simulink model "sk_QR_Balanced"  (Simulink 9.0)
settings: Solver=ode45  StartTime=0.0  StopTime=T_sim  MaxStep=1e-3  RelTol=1e-3  EnableMultiTasking=on
values from neighbouring files (symbols this model uses):
  Tm = 1e-3    (= 0.001)    [Ejecucion.m]
settings Model: Creator=Isa  LastModifiedBy=Raúl  ExtModeTrigMode=oneshot  ExtModeArmWhenConnect=off
settings DataIOCC: SignalLoggingSaveFormat=ModelDataLogs
settings OptimizationCC: BlockReduction=off  BooleanDataType=off  ExpressionDepthLimit=2147483647  InitFltsAndDblsToZero=on
settings DebuggingCC: SaveWithParameterizedLinksMsg=none  SignalResolutionControl=TryResolveAllWithWarning  MultiTaskDSMMsg=warning  MultiTaskCondExecSysMsg=none  FcnCallInpInsideContextMsg=warning  StateNameClashWarn=warning
settings HardwareCC: TargetUnknown=on
settings GRTTargetCC: TargetFcnLib=ansi_tfl_tmw.mat  GeneratePreprocessorConditionals=Disable all  CombineOutputUpdateFcns=off  GRTInterface=on
settings ConfigComp: CovSFcnEnable=off

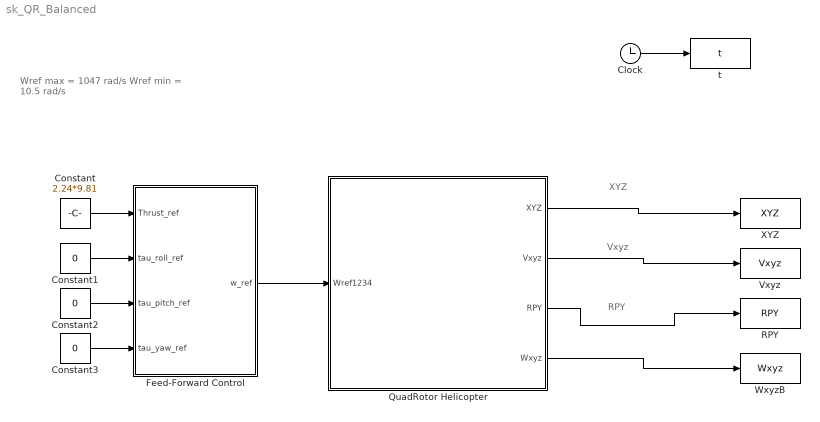
== system sk_QR_Balanced ==
  note: XYZ
  note: Vxyz
  note: RPY
  note: Wref max = 1047 rad/s
      | Wref min = 10.5 rad/s
  Clock : Clock
  Constant : Constant  Value=2.24*9.81
  Constant1 : Constant  Value=0
  Constant2 : Constant  Value=0
  Constant3 : Constant  Value=0
  Feed-Forward Control : Subsystem
  QuadRotor Helicopter : Subsystem  mask(Balanced Quadrotor Helicopter){X_ini=0, Y_ini=0, Z_ini=0}
      mask prompts: X_ini "X inicial (m)"; Y_ini "Y inicial (m)"; Z_ini "Z inicial (m)"
      mask help: Inputs: speed reference for each rotor.
      mask Display:
      | image(imread('QR.JPG'));
      | port_label('output', 1, 'XYZ');
      | port_label('output', 2, 'Vxyz');
      | port_label('output', 3, 'RPY');
      | port_label('output', 4, 'Wxyz');
      | port_label('input', 1, 'Wmref')
  RPY : ToWorkspace  VariableName=RPY  SampleTime=-1
  Vxyz : ToWorkspace  VariableName=Vxyz  SampleTime=-1
  WxyzB : ToWorkspace  VariableName=Wxyz  SampleTime=-1
  XYZ : ToWorkspace  VariableName=XYZ  SampleTime=-1
  t : ToWorkspace  VariableName=t  SampleTime=-1
  wires:
  Clock/1 -> t/1
  QuadRotor Helicopter/1(XYZ) -> XYZ/1
  QuadRotor Helicopter/3(RPY) -> RPY/1
  QuadRotor Helicopter/2(Vxyz) -> Vxyz/1
  QuadRotor Helicopter/4(Wxyz) -> WxyzB/1
  Feed-Forward Control/1(w_ref) -> QuadRotor Helicopter/1(Wref1234)
  Constant/1 -> Feed-Forward Control/1(Thrust_ref)
  Constant1/1 -> Feed-Forward Control/2(tau_roll_ref)
  Constant2/1 -> Feed-Forward Control/3(tau_pitch_ref)
  Constant3/1 -> Feed-Forward Control/4(tau_yaw_ref)

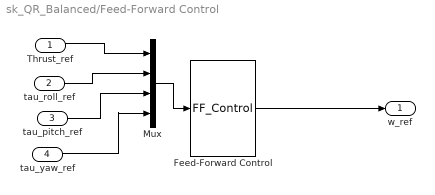
== system sk_QR_Balanced/Feed-Forward Control ==
  Thrust_ref : Inport
  tau_roll_ref : Inport  Port=2
  tau_pitch_ref : Inport  Port=3
  tau_yaw_ref : Inport  Port=4
  Feed-Forward Control : MATLABFcn  MATLABFcn=FF_Control  SampleTime=Tm
  Mux : Mux
  w_ref : Outport
  wires:
  Feed-Forward Control/1 -> w_ref/1
  Mux/1 -> Feed-Forward Control/1
  tau_roll_ref/1 -> Mux/2
  tau_yaw_ref/1 -> Mux/4
  tau_pitch_ref/1 -> Mux/3
  Thrust_ref/1 -> Mux/1

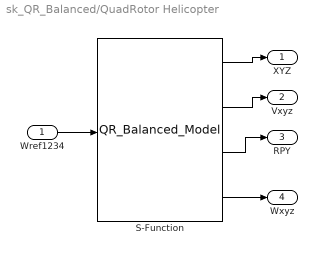
== system sk_QR_Balanced/QuadRotor Helicopter ==
  Wref1234 : Inport
  S-Function : S-Function  FunctionName=QR_Balanced_Model  Parameters=[X_ini, Y_ini, Z_ini]  SFunctionDeploymentMode=off  EnableBusSupport=off
  XYZ : Outport
  Vxyz : Outport  Port=2
  RPY : Outport  Port=3
  Wxyz : Outport  Port=4
  wires:
  Wref1234/1 -> S-Function/1
  S-Function/1 -> XYZ/1
  S-Function/2 -> Vxyz/1
  S-Function/3 -> RPY/1
  S-Function/4 -> Wxyz/1
